simulink model "Model"  (R2019b)
settings: Solver=VariableStepAuto  StartTime=0.0  StopTime=1000  RelTol=1e-3
values from neighbouring files (symbols this model uses):
  a_pow = 3    [Model_Run.m]
  C = 1    [Model_Run.m]
  c_pow = 3    [Model_Run.m]
  Cdiss = 10E-6    (= 1e-05)    [Model_Run.m]
  E_k = -75    [Model_Run.m]
  E_na = 35    [Model_Run.m]
  G_a = 36    [Model_Run.m]
  G_bar_ca = 2    [Model_Run.m]
  G_k = 12    [Model_Run.m]
  G_na = 40    [Model_Run.m]
  GkCa_Bar = .05    (= 0.05)    [Model_Run.m]
  H_init = 1    [Model_Run.m]
  I_stim = 1    [Model_Run.m]
  M_init = 0.0    (= 0)    [Model_Run.m]
  m_pow = 3    [Model_Run.m]
  N_init = 0.00    (= 0)    [Model_Run.m]
  n_pow = 4    [Model_Run.m]
  V_init = -62    [Model_Run.m]
  Zca = 2    [Model_Run.m]
undefined symbols (not defined in the file or in its folder): T_stim_start, T_stim_stop
settings Model: Creator=PranavM  LastModifiedBy=PranavM

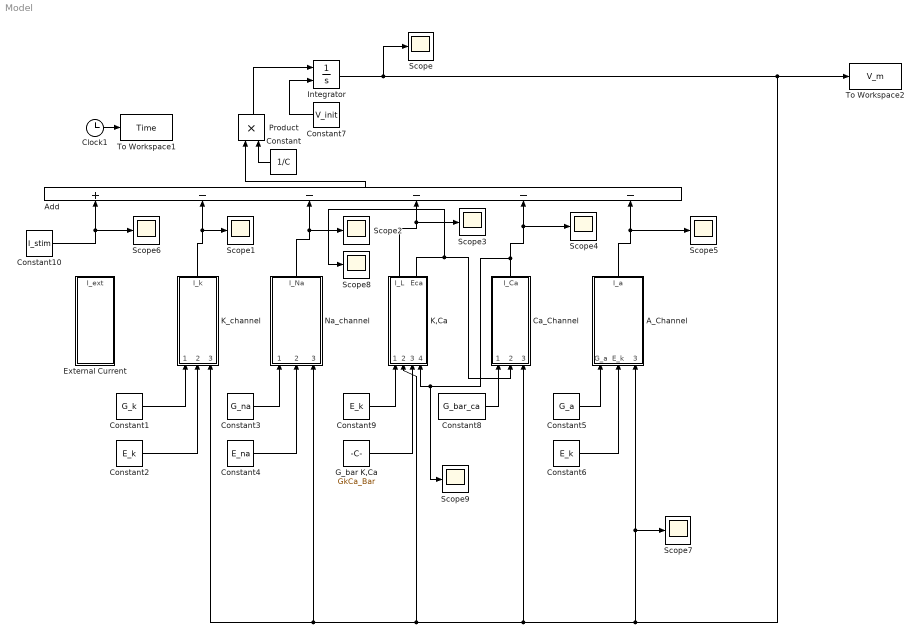
== system Model ==
  A_Channel : Subsystem
  Add : Sum  Inputs=+-----
  Ca_Channel : Subsystem
  Clock1 : Clock
  Constant : Constant  Value=1/C
  Constant1 : Constant  Value=G_k
  Constant10 : Constant  Value=I_stim
  Constant2 : Constant  Value=E_k
  Constant3 : Constant  Value=G_na
  Constant4 : Constant  Value=E_na
  Constant5 : Constant  Value=G_a
  Constant6 : Constant  Value=E_k
  Constant7 : Constant  Value=V_init
  Constant8 : Constant  Value=G_bar_ca
  Constant9 : Constant  Value=E_k
  External Current : Subsystem
  G_bar K,Ca : Constant  Value=GkCa_Bar
  Integrator : Integrator  InitialConditionSource=external
  K,Ca : Subsystem
  K_channel : Subsystem
  Na_channel : Subsystem
  Product : Product
  Scope{,1..9} (10 alike) : Scope
  To Workspace1 : ToWorkspace  VariableName=Time  SampleTime=-1
  To Workspace2 : ToWorkspace  VariableName=V_m  SampleTime=-1
  wires:
  Constant/1 -> Product/2
  Constant7/1 -> Integrator/2
  Clock1/1 -> To Workspace1/1
  Add/1 -> Product/1
  K_channel/1(I_k) -> Scope1/1, Add/2
  Na_channel/1(I_Na) -> Scope2/1, Add/3
  Ca_Channel/1(I_Ca) -> Scope9/1, K,Ca/4(Ica), Add/5, Scope4/1
  A_Channel/1(I_a) -> Scope5/1, Add/6
  K,Ca/2(Eca) -> Scope8/1, Ca_Channel/2(E_Ca)
  K,Ca/1(I_L) -> Add/4, Scope3/1
  Integrator/1 -> Ca_Channel/3(V_m), K,Ca/2(V_m), Na_channel/3(V_m), K_channel/3(V_m), Scope7/1, A_Channel/3(V_m), To Workspace2/1, Scope/1
  Constant1/1 -> K_channel/1(G_k)
  Constant2/1 -> K_channel/2(E_k)
  Constant4/1 -> Na_channel/2(E_na)
  Constant3/1 -> Na_channel/1(G_na)
  Constant6/1 -> A_Channel/2(E_k)
  Constant5/1 -> A_Channel/1(G_a)
  Constant8/1 -> Ca_Channel/1(G_bar_ca)
  Constant9/1 -> K,Ca/1(E_K)
  G_bar K,Ca/1 -> K,Ca/3(G_bar_k_ca)
  Product/1 -> Integrator/1
  Constant10/1 -> Scope6/1, Add/1

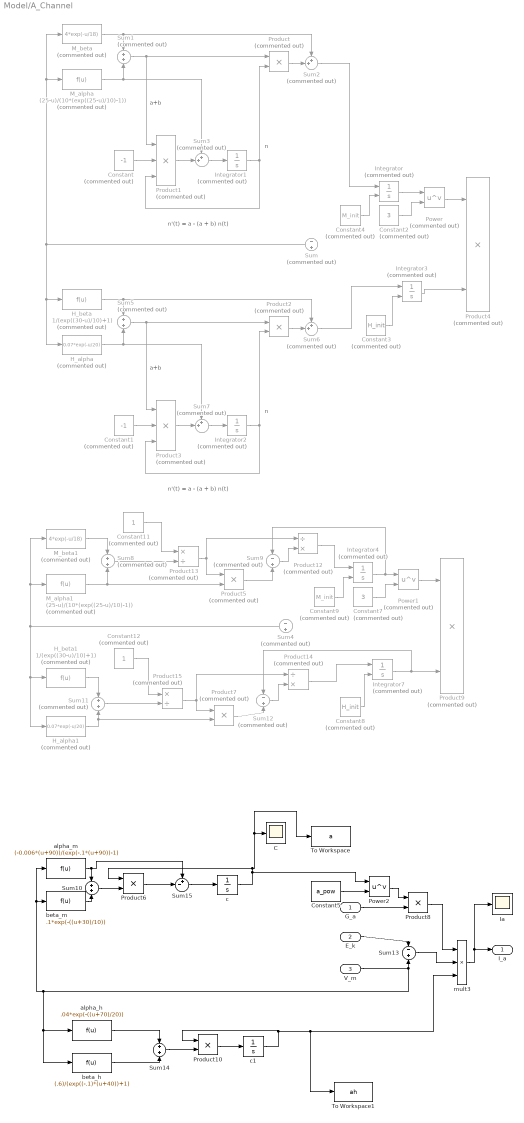
== system Model/A_Channel ==
  note: a+b
  note: n'(t) = a - (a + b) n(t)
  note: n
  note: n'(t) = a - (a + b) n(t)
  note: a+b
  note: n
  G_a : Inport
  E_k : Inport  Port=2
  V_m : Inport  Port=3
  C : Scope
  Constant : Constant  Commented=on  Value=-1
  Constant1 : Constant  Commented=on  Value=-1
  Constant11 : Constant  Commented=on
  Constant12 : Constant  Commented=on
  Constant2 : Constant  Commented=on  Value=3
  Constant3 : Constant  Commented=on  Value=H_init
  Constant4 : Constant  Commented=on  Value=M_init
  Constant5 : Constant  Value=a_pow
  Constant7 : Constant  Commented=on  Value=3
  Constant8 : Constant  Commented=on  Value=H_init
  Constant9 : Constant  Commented=on  Value=M_init
  H_alpha : Fcn  Commented=on  Expr=0.07*exp(-u/20)
  H_alpha1 : Fcn  Commented=on  Expr=0.07*exp(-u/20)
  H_beta : Fcn  Commented=on  Expr=1/(exp((30-u)/10)+1)
  H_beta1 : Fcn  Commented=on  Expr=1/(exp((30-u)/10)+1)
  Ia : Scope
  Integrator{,3..4,7} (4 alike) : Integrator  Commented=on  InitialConditionSource=external
  Integrator1 : Integrator  Commented=on
  Integrator2 : Integrator  Commented=on
  M_alpha : Fcn  Commented=on  Expr=(25-u)/(10*(exp((25-u)/10)-1))
  M_alpha1 : Fcn  Commented=on  Expr=(25-u)/(10*(exp((25-u)/10)-1))
  M_beta : Fcn  Commented=on  Expr=4*exp(-u/18)
  M_beta1 : Fcn  Commented=on  Expr=4*exp(-u/18)
  Power : Math  Commented=on  Operator=pow  SaturateOnIntegerOverflow=on
  Power1 : Math  Commented=on  Operator=pow  SaturateOnIntegerOverflow=on
  Power2 : Math  Operator=pow  SaturateOnIntegerOverflow=on
  Product{,2,5,7} (4 alike) : Product  Commented=on
  Product{1,3..4,9} (4 alike) : Product  Commented=on  Inputs=3
  Product10 : Product
  Product12 : Product  Commented=on  Inputs=/*
  Product13 : Product  Commented=on  Inputs=*/
  Product14 : Product  Commented=on  Inputs=/*
  Product15 : Product  Commented=on  Inputs=*/
  Product6 : Product
  Product8 : Product
  Sum{,4,9,12} (4 alike) : Sum  Commented=on  Inputs=-+
  Sum{1,5,8,11} (4 alike) : Sum  Commented=on
  Sum10 : Sum  Inputs=+|+
  Sum13 : Sum  Inputs=-+
  Sum14 : Sum  Inputs=+|+
  Sum15 : Sum  Inputs=+-|
  Sum{2..3,6..7} (4 alike) : Sum  Commented=on  Inputs=++|
  To Workspace : ToWorkspace  VariableName=a  SampleTime=-1
  To Workspace1 : ToWorkspace  VariableName=ah  SampleTime=-1
  alpha_h : Fcn  Expr=.04*exp(-((u+70)/20))
  alpha_m : Fcn  Expr=(-0.006*(u+90))/(exp(-.1*(u+90))-1)
  beta_h : Fcn  Expr=(.6)/(exp((-.1)*(u+40))+1)
  beta_m : Fcn  Expr=.1*exp(-((u+30)/10))
  c : Integrator
  c1 : Integrator
  mult3 : Product  Inputs=***
  I_a : Outport  VectorParamsAs1DForOutWhenUnconnected=off
  wires:
  M_beta/1 -> Sum2/1, Sum1/1
  Sum/1 -> M_beta/1, M_alpha/1, H_alpha/1, H_beta/1
  M_alpha/1 -> Sum3/1, Sum1/2
  Sum1/1 -> Product1/1, Product/1
  Constant/1 -> Product1/2
  Sum3/1 -> Integrator1/1
  Integrator1/1 -> Product/2, Product1/3
  Product/1 -> Sum2/2
  Product1/1 -> Sum3/2
  Sum7/1 -> Integrator2/1
  Product3/1 -> Sum7/2
  Integrator2/1 -> Product2/2, Product3/3
  Product2/1 -> Sum6/2
  Constant1/1 -> Product3/2
  Sum5/1 -> Product3/1, Product2/1
  H_beta/1 -> Sum6/1, Sum5/1
  H_alpha/1 -> Sum7/1, Sum5/2
  Constant2/1 -> Power/2
  Integrator/1 -> Power/1
  Sum2/1 -> Integrator/1
  Power/1 -> Product4/1
  Integrator3/1 -> Product4/3
  Sum6/1 -> Integrator3/1
  Constant3/1 -> Integrator3/2
  Constant4/1 -> Integrator/2
  Constant8/1 -> Integrator7/2
  M_beta1/1 -> Sum8/1
  Integrator4/1 -> Sum9/1, Power1/1
  H_beta1/1 -> Sum11/1
  Power1/1 -> Product9/1
  Sum4/1 -> H_alpha1/1, H_beta1/1, M_beta1/1, M_alpha1/1
  Constant9/1 -> Integrator4/2
  Integrator7/1 -> Sum12/1, Product9/3
  Constant7/1 -> Power1/2
  Product13/1 -> Product5/1, Product12/1
  M_alpha1/1 -> Product5/2, Sum8/2
  Product5/1 -> Sum9/2
  Constant11/1 -> Product13/1
  Product12/1 -> Integrator4/1
  Sum9/1 -> Product12/2
  Sum8/1 -> Product13/2
  Product15/1 -> Product14/1, Product7/1
  H_alpha1/1 -> Product7/2, Sum11/2
  Product7/1 -> Sum12/2
  Constant12/1 -> Product15/1
  Sum12/1 -> Product14/2
  Sum11/1 -> Product15/2
  Product14/1 -> Integrator7/1
  c/1 -> To Workspace/1, C/1, Product6/1, Power2/1
  alpha_m/1 -> Sum15/1, Sum10/1
  beta_m/1 -> Sum10/2
  G_a/1 -> Product8/2
  E_k/1 -> Sum13/1
  Sum13/1 -> mult3/2
  Constant5/1 -> Power2/2
  Product8/1 -> mult3/1
  Power2/1 -> Product8/1
  mult3/1 -> Ia/1, I_a/1
  Product10/1 -> c1/1
  beta_h/1 -> Sum14/2
  V_m/1 -> Sum13/2, beta_m/1, alpha_m/1, beta_h/1, alpha_h/1
  alpha_h/1 -> Sum14/1
  Sum14/1 -> Product10/2
  c1/1 -> To Workspace1/1, mult3/3, Product10/1
  Sum10/1 -> Product6/2
  Product6/1 -> Sum15/2
  Sum15/1 -> c/1

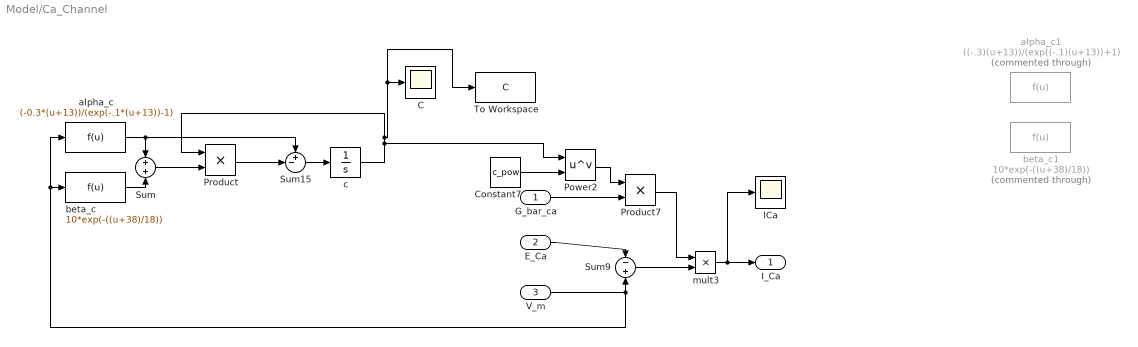
== system Model/Ca_Channel ==
  G_bar_ca : Inport
  E_Ca : Inport  Port=2
  V_m : Inport  Port=3
  C : Scope
  Constant7 : Constant  Value=c_pow
  ICa : Scope
  Power2 : Math  Operator=pow  SaturateOnIntegerOverflow=on
  Product : Product
  Product7 : Product
  Sum : Sum  Inputs=+|+
  Sum15 : Sum  Inputs=+-|
  Sum9 : Sum  Inputs=-+
  To Workspace : ToWorkspace  VariableName=C  SampleTime=-1
  alpha_c : Fcn  Expr=(-0.3*(u+13))/(exp(-.1*(u+13))-1)
  alpha_c1 : Fcn  Commented=through  Expr=((-.3)(u+13))/(exp((-.1)(u+13))+1)
  beta_c : Fcn  Expr=10*exp(-((u+38)/18))
  beta_c1 : Fcn  Commented=through  Expr=10*exp(-((u+38)/18))
  c : Integrator
  mult3 : Product  Inputs=**
  I_Ca : Outport  VectorParamsAs1DForOutWhenUnconnected=off
  wires:
  Power2/1 -> Product7/1
  c/1 -> Product/1, To Workspace/1, C/1, Power2/1
  Product7/1 -> mult3/1
  mult3/1 -> ICa/1, I_Ca/1
  Sum9/1 -> mult3/2
  Constant7/1 -> Power2/2
  V_m/1 -> Sum9/2, alpha_c/1, beta_c/1
  E_Ca/1 -> Sum9/1
  G_bar_ca/1 -> Product7/2
  alpha_c/1 -> Sum15/1, Sum/1
  beta_c/1 -> Sum/2
  Sum/1 -> Product/2
  Product/1 -> Sum15/2
  Sum15/1 -> c/1

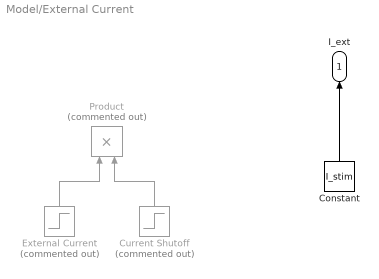
== system Model/External Current ==
  Constant : Constant  Value=I_stim
  Current Shutoff : Step  Commented=on  Time=T_stim_stop  Before=1  After=0  SampleTime=0
  External Current : Step  Commented=on  Time=T_stim_start  After=I_stim  SampleTime=0
  Product : Product  Commented=on
  I_ext : Outport  VectorParamsAs1DForOutWhenUnconnected=off
  wires:
  External Current/1 -> Product/1
  Current Shutoff/1 -> Product/2
  Constant/1 -> I_ext/1

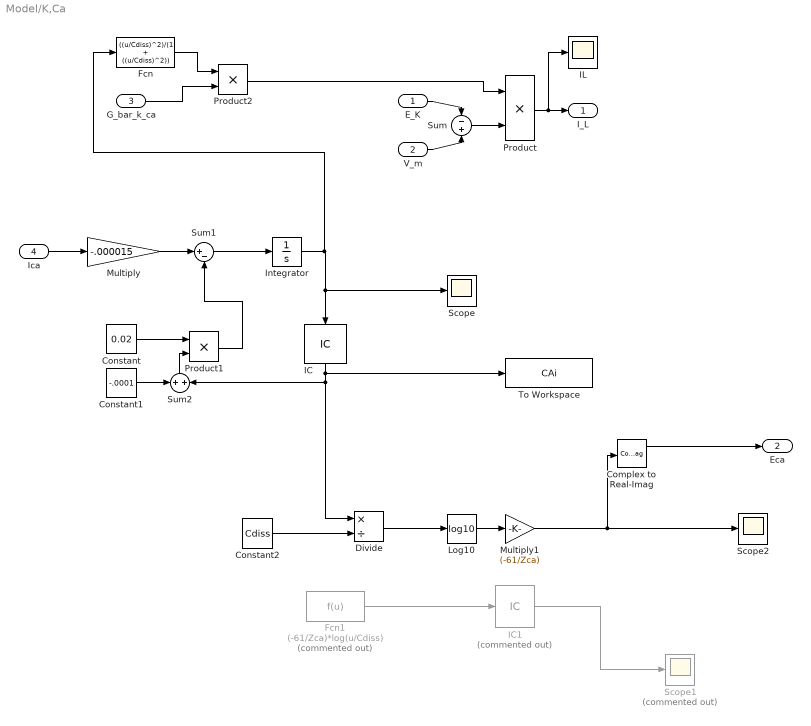
== system Model/K,Ca ==
  E_K : Inport
  V_m : Inport  Port=2
  G_bar_k_ca : Inport  Port=3
  Ica : Inport  Port=4
  Complex to Real-Imag : ComplexToRealImag
  Constant : Constant  Value=0.02
  Constant1 : Constant  Value=-.0001
  Constant2 : Constant  Value=Cdiss
  Divide : Product  Inputs=*/
  Fcn : Fcn  Expr=((u/Cdiss)^2)/(1 + ((u/Cdiss)^2))
  Fcn1 : Fcn  Commented=on  Expr=(-61/Zca)*log(u/Cdiss)
  IC : InitialCondition  Value=10E-7
  IC1 : InitialCondition  Commented=on
  IL : Scope
  Integrator : Integrator
  Log10 : Math  Operator=log10  SignedPower=off  SaturateOnIntegerOverflow=on
  Multiply : Gain  Gain=-.000015
  Multiply1 : Gain  Gain=(-61/Zca)
  Product : Product
  Product1 : Product
  Product2 : Product
  Scope : Scope
  Scope1 : Scope  Commented=on
  Scope2 : Scope
  Sum : Sum  Inputs=-+
  Sum1 : Sum  Inputs=|+-
  Sum2 : Sum
  To Workspace : ToWorkspace  VariableName=CAi  SampleTime=-1
  I_L : Outport  VectorParamsAs1DForOutWhenUnconnected=off
  Eca : Outport  Port=2
  wires:
  Ica/1 -> Multiply/1
  Multiply/1 -> Sum1/1
  Sum1/1 -> Integrator/1
  Constant1/1 -> Sum2/1
  Integrator/1 -> Scope/1, IC/1, Fcn/1
  Sum2/1 -> Product1/2
  Constant/1 -> Product1/1
  Product1/1 -> Sum1/2
  G_bar_k_ca/1 -> Product2/2
  Fcn/1 -> Product2/1
  Product/1 -> IL/1, I_L/1
  Sum/1 -> Product/2
  E_K/1 -> Sum/1
  V_m/1 -> Sum/2
  Product2/1 -> Product/1
  IC/1 -> To Workspace/1, Divide/1, Sum2/2
  Fcn1/1 -> IC1/1
  IC1/1 -> Scope1/1
  Divide/1 -> Log10/1
  Multiply1/1 -> Complex to Real-Imag/1, Scope2/1
  Constant2/1 -> Divide/2
  Complex to Real-Imag/1 -> Eca/1
  Log10/1 -> Multiply1/1

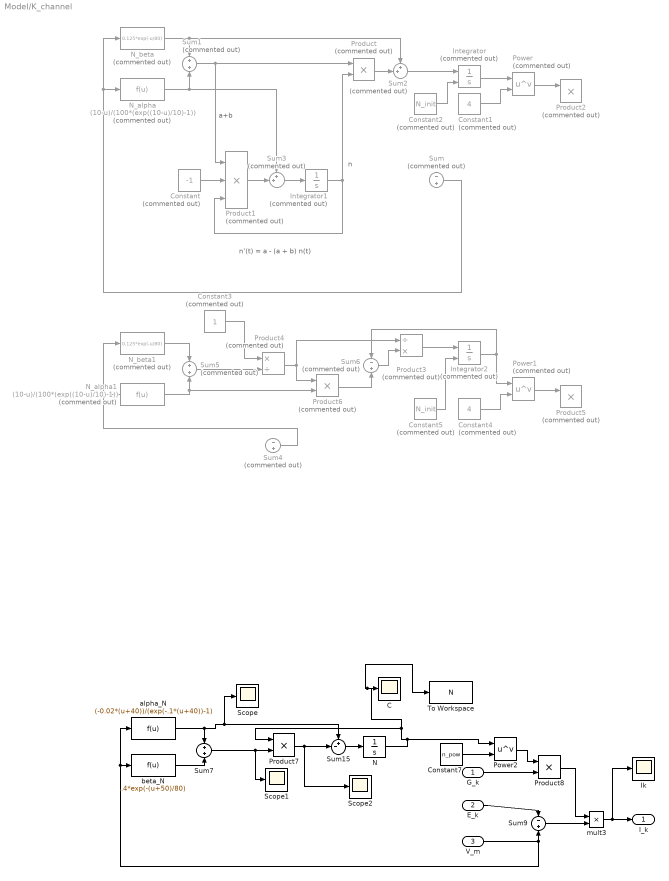
== system Model/K_channel ==
  note: a+b
  note: n
  note: n'(t) = a - (a + b) n(t)
  G_k : Inport
  E_k : Inport  Port=2
  V_m : Inport  Port=3
  C : Scope
  Constant : Constant  Commented=on  Value=-1
  Constant1 : Constant  Commented=on  Value=4
  Constant2 : Constant  Commented=on  Value=N_init
  Constant3 : Constant  Commented=on
  Constant4 : Constant  Commented=on  Value=4
  Constant5 : Constant  Commented=on  Value=N_init
  Constant7 : Constant  Value=n_pow
  Ik : Scope
  Integrator : Integrator  Commented=on  InitialConditionSource=external
  Integrator1 : Integrator  Commented=on
  Integrator2 : Integrator  Commented=on  InitialConditionSource=external
  N : Integrator
  N_alpha : Fcn  Commented=on  Expr=(10-u)/(100*(exp((10-u)/10)-1))
  N_alpha1 : Fcn  Commented=on  Expr=(10-u)/(100*(exp((10-u)/10)-1))
  N_beta : Fcn  Commented=on  Expr=0.125*exp(-u/80)
  N_beta1 : Fcn  Commented=on  Expr=0.125*exp(-u/80)
  Power : Math  Commented=on  Operator=pow  SaturateOnIntegerOverflow=on
  Power1 : Math  Commented=on  Operator=pow  SaturateOnIntegerOverflow=on
  Power2 : Math  Operator=pow  SaturateOnIntegerOverflow=on
  Product{,2,5..6} (4 alike) : Product  Commented=on
  Product1 : Product  Commented=on  Inputs=3
  Product3 : Product  Commented=on  Inputs=/*
  Product4 : Product  Commented=on  Inputs=*/
  Product7 : Product
  Product8 : Product
  Scope : Scope
  Scope1 : Scope
  Scope2 : Scope
  Sum : Sum  Commented=on  Inputs=-+
  Sum1 : Sum  Commented=on
  Sum15 : Sum  Inputs=+-|
  Sum2 : Sum  Commented=on  Inputs=++|
  Sum3 : Sum  Commented=on  Inputs=++|
  Sum4 : Sum  Commented=on  Inputs=-+
  Sum5 : Sum  Commented=on
  Sum6 : Sum  Commented=on  Inputs=-+
  Sum7 : Sum  Inputs=+|+
  Sum9 : Sum  Inputs=-+
  To Workspace : ToWorkspace  VariableName=N  SampleTime=-1
  alpha_N : Fcn  Expr=(-0.02*(u+40))/(exp(-.1*(u+40))-1)
  beta_N : Fcn  Expr=.4*exp(-(u+50)/80)
  mult3 : Product  Inputs=**
  I_k : Outport  VectorParamsAs1DForOutWhenUnconnected=off
  wires:
  N_beta/1 -> Sum2/1, Sum1/1
  N_alpha/1 -> Sum3/1, Sum1/2
  Product/1 -> Sum2/2
  Sum2/1 -> Integrator/1
  Sum1/1 -> Product1/1, Product/1
  Constant/1 -> Product1/2
  Product1/1 -> Sum3/2
  Sum3/1 -> Integrator1/1
  Integrator1/1 -> Product/2, Product1/3
  Integrator/1 -> Power/1
  Constant1/1 -> Power/2
  Power/1 -> Product2/1
  Sum/1 -> N_beta/1, N_alpha/1
  Constant2/1 -> Integrator/2
  Sum4/1 -> N_alpha1/1, N_beta1/1
  Power1/1 -> Product5/1
  N_alpha1/1 -> Product6/2, Sum5/2
  Integrator2/1 -> Power1/1, Sum6/1
  N_beta1/1 -> Sum5/1
  Constant5/1 -> Integrator2/2
  Constant4/1 -> Power1/2
  Sum5/1 -> Product4/2
  Constant3/1 -> Product4/1
  Product4/1 -> Product3/1, Product6/1
  Product6/1 -> Sum6/2
  Sum6/1 -> Product3/2
  Product3/1 -> Integrator2/1
  N/1 -> To Workspace/1, C/1, Product7/1, Power2/1
  alpha_N/1 -> Scope/1, Sum15/1, Sum7/1
  beta_N/1 -> Sum7/2
  G_k/1 -> Product8/2
  V_m/1 -> Sum9/2, beta_N/1, alpha_N/1
  E_k/1 -> Sum9/1
  Sum9/1 -> mult3/2
  Constant7/1 -> Power2/2
  Product8/1 -> mult3/1
  Power2/1 -> Product8/1
  mult3/1 -> Ik/1, I_k/1
  Product7/1 -> Sum15/2, Scope2/1
  Sum7/1 -> Scope1/1, Product7/2
  Sum15/1 -> N/1

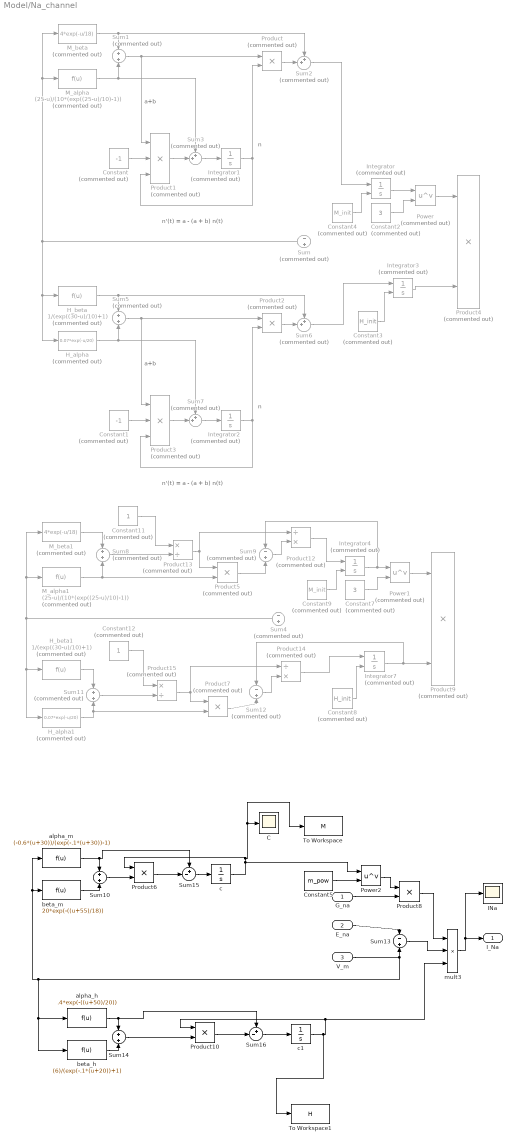
== system Model/Na_channel ==
  note: a+b
  note: n'(t) = a - (a + b) n(t)
  note: n
  note: n'(t) = a - (a + b) n(t)
  note: a+b
  note: n
  G_na : Inport
  E_na : Inport  Port=2
  V_m : Inport  Port=3
  C : Scope
  Constant : Constant  Commented=on  Value=-1
  Constant1 : Constant  Commented=on  Value=-1
  Constant11 : Constant  Commented=on
  Constant12 : Constant  Commented=on
  Constant2 : Constant  Commented=on  Value=3
  Constant3 : Constant  Commented=on  Value=H_init
  Constant4 : Constant  Commented=on  Value=M_init
  Constant5 : Constant  Value=m_pow
  Constant7 : Constant  Commented=on  Value=3
  Constant8 : Constant  Commented=on  Value=H_init
  Constant9 : Constant  Commented=on  Value=M_init
  H_alpha : Fcn  Commented=on  Expr=0.07*exp(-u/20)
  H_alpha1 : Fcn  Commented=on  Expr=0.07*exp(-u/20)
  H_beta : Fcn  Commented=on  Expr=1/(exp((30-u)/10)+1)
  H_beta1 : Fcn  Commented=on  Expr=1/(exp((30-u)/10)+1)
  INa : Scope
  Integrator{,3..4,7} (4 alike) : Integrator  Commented=on  InitialConditionSource=external
  Integrator1 : Integrator  Commented=on
  Integrator2 : Integrator  Commented=on
  M_alpha : Fcn  Commented=on  Expr=(25-u)/(10*(exp((25-u)/10)-1))
  M_alpha1 : Fcn  Commented=on  Expr=(25-u)/(10*(exp((25-u)/10)-1))
  M_beta : Fcn  Commented=on  Expr=4*exp(-u/18)
  M_beta1 : Fcn  Commented=on  Expr=4*exp(-u/18)
  Power : Math  Commented=on  Operator=pow  SaturateOnIntegerOverflow=on
  Power1 : Math  Commented=on  Operator=pow  SaturateOnIntegerOverflow=on
  Power2 : Math  Operator=pow  SaturateOnIntegerOverflow=on
  Product{,2,5,7} (4 alike) : Product  Commented=on
  Product{1,3..4,9} (4 alike) : Product  Commented=on  Inputs=3
  Product10 : Product
  Product12 : Product  Commented=on  Inputs=/*
  Product13 : Product  Commented=on  Inputs=*/
  Product14 : Product  Commented=on  Inputs=/*
  Product15 : Product  Commented=on  Inputs=*/
  Product6 : Product
  Product8 : Product
  Sum{,4,9,12} (4 alike) : Sum  Commented=on  Inputs=-+
  Sum{1,5,8,11} (4 alike) : Sum  Commented=on
  Sum10 : Sum  Inputs=+|+
  Sum13 : Sum  Inputs=-+
  Sum14 : Sum  Inputs=+|+
  Sum15 : Sum  Inputs=+-|
  Sum16 : Sum  Inputs=+-|
  Sum{2..3,6..7} (4 alike) : Sum  Commented=on  Inputs=++|
  To Workspace : ToWorkspace  VariableName=M  SampleTime=-1
  To Workspace1 : ToWorkspace  VariableName=H  SampleTime=-1
  alpha_h : Fcn  Expr=.4*exp(-((u+50)/20))
  alpha_m : Fcn  Expr=(-0.6*(u+30))/(exp(-.1*(u+30))-1)
  beta_h : Fcn  Expr=(6)/(exp(-.1*(u+20))+1)
  beta_m : Fcn  Expr=20*exp(-((u+55)/18))
  c : Integrator
  c1 : Integrator
  mult3 : Product  Inputs=***
  I_Na : Outport  VectorParamsAs1DForOutWhenUnconnected=off
  wires:
  M_beta/1 -> Sum2/1, Sum1/1
  Sum/1 -> M_beta/1, M_alpha/1, H_alpha/1, H_beta/1
  M_alpha/1 -> Sum3/1, Sum1/2
  Sum1/1 -> Product1/1, Product/1
  Constant/1 -> Product1/2
  Sum3/1 -> Integrator1/1
  Integrator1/1 -> Product/2, Product1/3
  Product/1 -> Sum2/2
  Product1/1 -> Sum3/2
  Sum7/1 -> Integrator2/1
  Product3/1 -> Sum7/2
  Integrator2/1 -> Product2/2, Product3/3
  Product2/1 -> Sum6/2
  Constant1/1 -> Product3/2
  Sum5/1 -> Product3/1, Product2/1
  H_beta/1 -> Sum6/1, Sum5/1
  H_alpha/1 -> Sum7/1, Sum5/2
  Constant2/1 -> Power/2
  Integrator/1 -> Power/1
  Sum2/1 -> Integrator/1
  Power/1 -> Product4/1
  Integrator3/1 -> Product4/3
  Sum6/1 -> Integrator3/1
  Constant3/1 -> Integrator3/2
  Constant4/1 -> Integrator/2
  Constant8/1 -> Integrator7/2
  M_beta1/1 -> Sum8/1
  Integrator4/1 -> Sum9/1, Power1/1
  H_beta1/1 -> Sum11/1
  Power1/1 -> Product9/1
  Sum4/1 -> H_alpha1/1, H_beta1/1, M_beta1/1, M_alpha1/1
  Constant9/1 -> Integrator4/2
  Integrator7/1 -> Sum12/1, Product9/3
  Constant7/1 -> Power1/2
  Product13/1 -> Product5/1, Product12/1
  M_alpha1/1 -> Product5/2, Sum8/2
  Product5/1 -> Sum9/2
  Constant11/1 -> Product13/1
  Product12/1 -> Integrator4/1
  Sum9/1 -> Product12/2
  Sum8/1 -> Product13/2
  Product15/1 -> Product14/1, Product7/1
  H_alpha1/1 -> Product7/2, Sum11/2
  Product7/1 -> Sum12/2
  Constant12/1 -> Product15/1
  Sum12/1 -> Product14/2
  Sum11/1 -> Product15/2
  Product14/1 -> Integrator7/1
  c/1 -> Product6/1, To Workspace/1, C/1, Power2/1
  alpha_m/1 -> Sum15/1, Sum10/1
  beta_m/1 -> Sum10/2
  G_na/1 -> Product8/2
  E_na/1 -> Sum13/1
  Sum13/1 -> mult3/2
  Constant5/1 -> Power2/2
  Product8/1 -> mult3/1
  Power2/1 -> Product8/1
  mult3/1 -> INa/1, I_Na/1
  beta_h/1 -> Sum14/2
  V_m/1 -> Sum13/2, beta_m/1, alpha_m/1, beta_h/1, alpha_h/1
  alpha_h/1 -> Sum16/1, Sum14/1
  c1/1 -> To Workspace1/1, Product10/1, mult3/3
  Sum10/1 -> Product6/2
  Product6/1 -> Sum15/2
  Sum14/1 -> Product10/2
  Sum16/1 -> c1/1
  Sum15/1 -> c/1
  Product10/1 -> Sum16/2
